simulink model "Subsystem"  (R2020b)
settings: Solver=VariableStepAuto  StartTime=0.0  StopTime=10.0  RelTol=1e-3
settings Model: Creator=shoun  LastModifiedBy=shoun
settings DataIOCC: SaveOutput=off  SaveTime=off

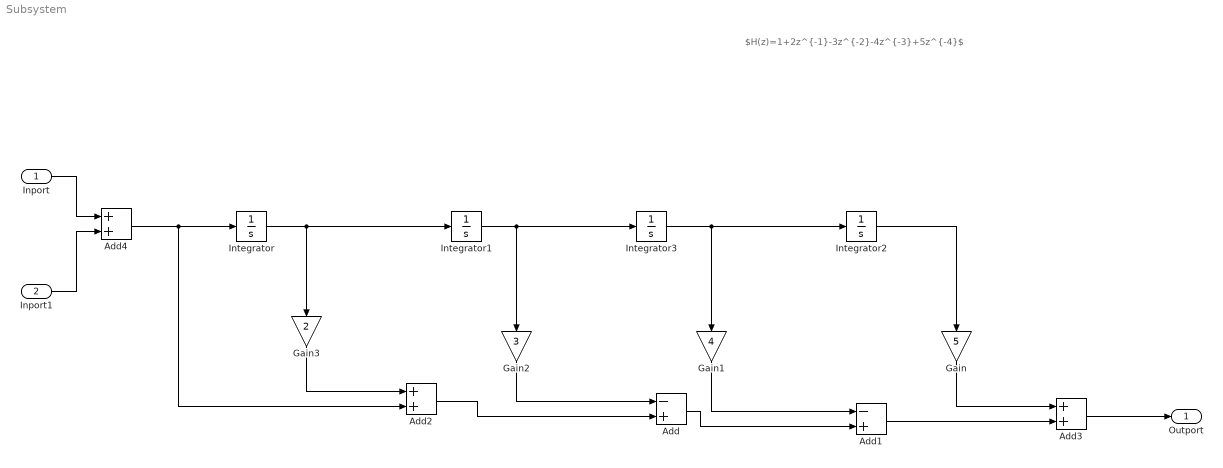
== system Subsystem ==
  note: $H(z)=1+2z^{-1}-3z^{-2}-4z^{-3}+5z^{-4}$
  Inport : Inport
  Inport1 : Inport  Port=2
  Add : Sum  Inputs=-+
  Add1 : Sum  Inputs=-+
  Add2 : Sum
  Add3 : Sum
  Add4 : Sum
  Gain : Gain  Gain=5
  Gain1 : Gain  Gain=4
  Gain2 : Gain  Gain=3
  Gain3 : Gain  Gain=2
  Integrator{,1..3} (4 alike) : Integrator
  Outport : Outport
  wires:
  Integrator3/1 -> Integrator2/1, Gain1/1
  Integrator1/1 -> Gain2/1, Integrator3/1
  Integrator/1 -> Integrator1/1, Gain3/1
  Inport1/1 -> Add4/2
  Add1/1 -> Add3/2
  Gain1/1 -> Add1/1
  Gain/1 -> Add3/1
  Integrator2/1 -> Gain/1
  Gain2/1 -> Add/1
  Add/1 -> Add1/2
  Inport/1 -> Add4/1
  Add4/1 -> Integrator/1, Add2/2
  Gain3/1 -> Add2/1
  Add2/1 -> Add/2
  Add3/1 -> Outport/1
